simulink model "inversor_no_ideal_SS"  (R2023b)
settings: Solver=VariableStepAuto  StartTime=0.0  StopTime=10.0  RelTol=1e-3
undefined symbols (not defined in the file or in its folder): A_v, B_v, C_v, D_v
settings Model: Creator=Pc  LastModifiedBy=Pc

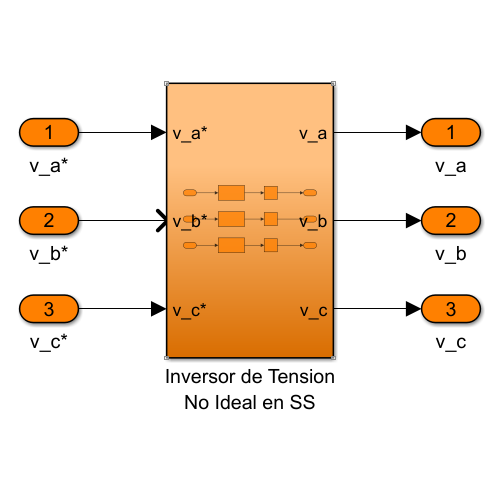
[thumbnail: Simulink's stored preview of the top-level diagram]
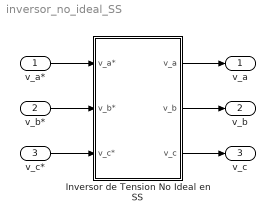
== system inversor_no_ideal_SS ==
  v_a* : Inport
  v_b* : Inport  Port=2
  v_c* : Inport  Port=3
  Inversor de Tension No Ideal en SS : Subsystem
  v_a : Outport
  v_b : Outport  Port=2
  v_c : Outport  Port=3
  wires:
  v_a*/1 -> Inversor de Tension No Ideal en SS/1(v_a*)
  v_b*/1 -> Inversor de Tension No Ideal en SS/2(v_b*)
  v_c*/1 -> Inversor de Tension No Ideal en SS/3(v_c*)
  Inversor de Tension No Ideal en SS/1(v_a) -> v_a/1
  Inversor de Tension No Ideal en SS/2(v_b) -> v_b/1
  Inversor de Tension No Ideal en SS/3(v_c) -> v_c/1

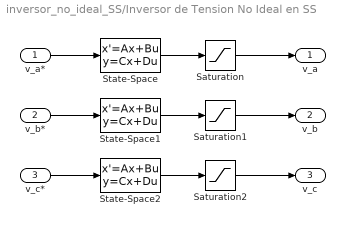
== system inversor_no_ideal_SS/Inversor de Tension No Ideal en SS ==
  v_a* : Inport
  v_b* : Inport  Port=2
  v_c* : Inport  Port=3
  Saturation : Saturate  UpperLimit=39.19  LowerLimit=-39.19
  Saturation1 : Saturate  UpperLimit=39.19  LowerLimit=-39.19
  Saturation2 : Saturate  UpperLimit=39.19  LowerLimit=-39.19
  State-Space : StateSpace  A=A_v  B=B_v  C=C_v  D=D_v  InitialCondition=0
  State-Space1 : StateSpace  A=A_v  B=B_v  C=C_v  D=D_v  InitialCondition=0
  State-Space2 : StateSpace  A=A_v  B=B_v  C=C_v  D=D_v  InitialCondition=0
  v_a : Outport
  v_b : Outport  Port=2
  v_c : Outport  Port=3
  wires:
  Saturation1/1 -> v_b/1
  State-Space1/1 -> Saturation1/1
  Saturation/1 -> v_a/1
  v_c*/1 -> State-Space2/1
  Saturation2/1 -> v_c/1
  State-Space2/1 -> Saturation2/1
  v_b*/1 -> State-Space1/1
  State-Space/1 -> Saturation/1
  v_a*/1 -> State-Space/1
